simulink model "mdl_lut"  (R2024a)
settings: Solver=ode45  StartTime=0.0  StopTime=STOP_T  RelTol=1e-3
values from neighbouring files (symbols this model uses):
  BP = evalin('base','BP')    [run_all.m]    (also in run_no_pso.m = linspace(-1,1,11); run_pso.m; run_verification.m; run_verify_and_convergence.m)
  STOP_T = 10    [run_no_pso.m]
  TBL = reshape(x, opt.tblSize)    [eval_lut_cost.m]    (also in run_all.m = evalin('base','TBL'); run_no_pso.m = zeros(size(BP)); run_verification.m = evalin('base','TBL'); run_verify_and_convergence.m = evalin('base','TBL'))
settings Model: Creator=mccat  LastModifiedBy=mccat
settings DataIOCC: SaveFormat=StructureWithTime

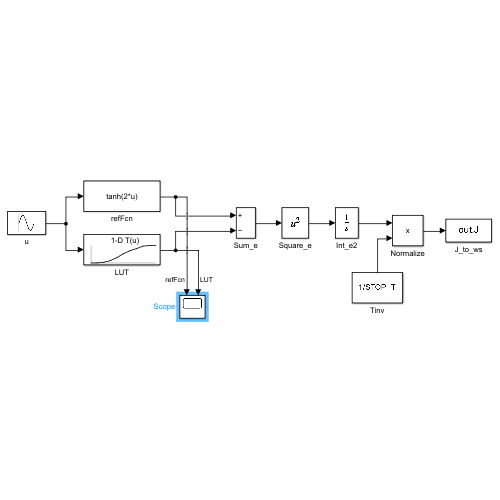
[thumbnail: Simulink's stored preview of the top-level diagram]
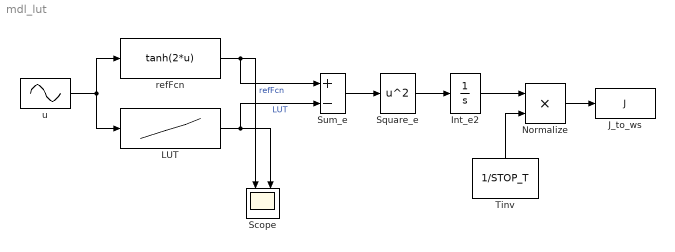
== system mdl_lut ==
  Int_e2 : Integrator
  J_to_ws : ToWorkspace  VariableName=J  SampleTime=-1
  LUT : Lookup_n-D  NumberOfTableDimensions=1  BreakpointsForDimension1=BP  Table=TBL  ExtrapMethod=Clip  InternalRulePriority=Speed  RndMeth=Simplest
  Normalize : Product  Inputs=**
  Scope : Scope  NumInputPorts=2
  Square_e : Math  Operator=square
  Sum_e : Sum  Inputs=+-
  Tinv : Constant  Value=1/STOP_T
  refFcn : Fcn  Expr=tanh(2*u)
  u : Sin  SampleTime=0
  wires:
  u/1 -> refFcn/1, LUT/1
  refFcn/1 -> Scope/1, Sum_e/1  "refFcn"
  LUT/1 -> Scope/2, Sum_e/2  "LUT"
  Sum_e/1 -> Square_e/1
  Square_e/1 -> Int_e2/1
  Int_e2/1 -> Normalize/1
  Tinv/1 -> Normalize/2
  Normalize/1 -> J_to_ws/1
